simulink model "imusim"  (R2015b)
settings: Solver=FixedStepAuto  StartTime=0.0  StopTime=100  FixedStep=Ts  RelTol=1e-3
values from neighbouring files (symbols this model uses):
  A = quat2mat(q)    [drawframe.m]
  s = sin(theta)    [Phi.m]    (also in ekf_sfun.m = sin(th))
  Ts = 1e-3    (= 0.001)    [setup.m]
undefined symbols (not defined in the file or in its folder): A2, B, B2, X, Y, Z
libraries: sm_lib x12, nesl_utility x8
settings Model: Creator=robots  LastModifiedBy=robots
settings DataIOCC: SaveFormat=Array
settings HardwareCC: ProdBitPerPointer=32  ProdLargestAtomicFloat=None  ProdIntDivRoundTo=Undefined  ProdEndianess=Unspecified  ProdWordSize=32  ProdHWDeviceType=32-bit Generic
settings GRTTargetCC: GeneratePreprocessorConditionals=Disable all
settings ConfigComp: CovModelRefEnable=Off

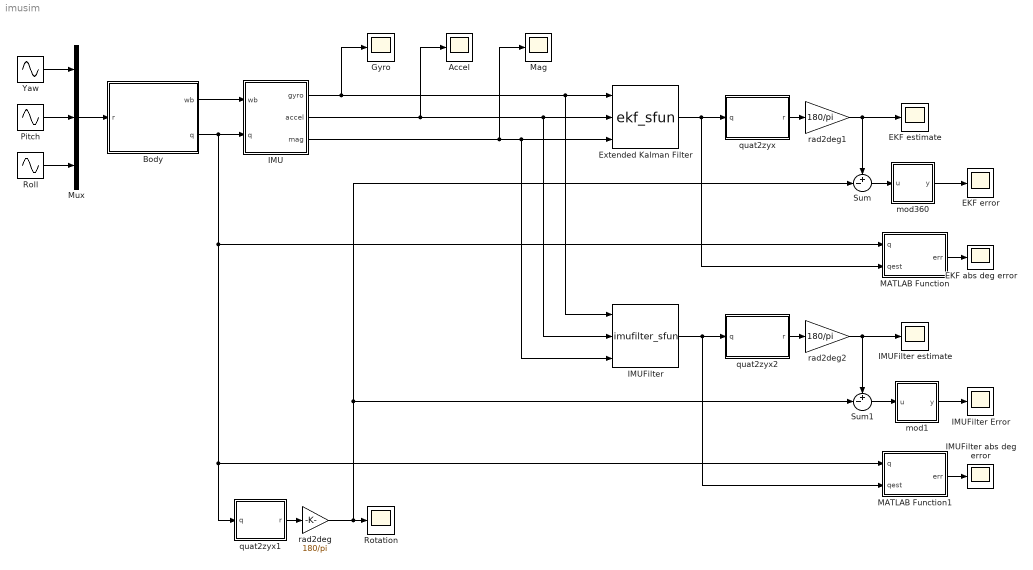
== system imusim ==
  Accel : Scope
  Body : Subsystem
  EKF abs deg error : Scope
  EKF error : Scope
  EKF estimate : Scope
  Extended Kalman Filter : M-S-Function  FunctionName=ekf_sfun  Parameters=Ts, Q, R, gs  mask{Ts=Ts, Q=diag([1 1 1 1]), R=diag([1e6*[1 1 1] 1e8*[1 1 1]]), gs=500/180*pi/2^15}
      mask prompts: Ts "Sample time (-1 for inherited):"; Q "Model covariance matrix (Q):"; R "Measurement covariance matrix (R):"; gs "Rate gyro scale:"
      mask Display:
      | port_label('input', 1, 'gyro')
      | port_label('input', 2, 'accel')
      | port_label('input', 3, 'mag')
      | port_label('output', 1, 'q')
  Gyro : Scope
  IMU : Subsystem
  IMUFilter : M-S-Function  FunctionName=imufilter_sfun  Parameters=Ts, gv, av, mv, gs  mask{Ts=Ts, gv=1, av=1e6, mv=1e8, gs=500/180*pi/2^15}
      mask prompts: Ts "Sample time (-1 for inherited):"; gv "Rate gyro variance:"; av "Accelerometer variance:"; mv "Magnetometer variance:"; gs "Rate gyro scale:"
      mask Display:
      | port_label('input', 1, 'gyro')
      | port_label('input', 2, 'accel')
      | port_label('input', 3, 'mag')
      | port_label('output', 1, 'q')
  IMUFilter abs deg error : Scope
  IMUFilter Error : Scope
  IMUFilter estimate : Scope
  MATLAB Function : MATLAB Function  TreatAsAtomicUnit=on
  MATLAB Function1 : MATLAB Function  TreatAsAtomicUnit=on
  Mag : Scope
  Mux : Mux  Inputs=3
  Pitch : Sin  Amplitude=0.5  Frequency=2*pi  SampleTime=0
  Roll : Sin  Amplitude=0  Frequency=2*pi  SampleTime=0
  Rotation : Scope
  Sum : Sum  Inputs=+-|
  Sum1 : Sum  Inputs=+-|
  Yaw : Sin  Amplitude=0  Frequency=2*pi  SampleTime=0
  mod1 : MATLAB Function  TreatAsAtomicUnit=on
  mod360 : MATLAB Function  TreatAsAtomicUnit=on
  quat2zyx : MATLAB Function  TreatAsAtomicUnit=on
  quat2zyx1 : MATLAB Function  TreatAsAtomicUnit=on
  quat2zyx2 : MATLAB Function  TreatAsAtomicUnit=on
  rad2deg : Gain  Gain=180/pi
  rad2deg1 : Gain  Gain=180/pi
  rad2deg2 : Gain  Gain=180/pi
  wires:
  Extended Kalman Filter/1 -> quat2zyx/1(q), MATLAB Function/2(qest)
  quat2zyx/1(r) -> rad2deg1/1
  Sum/1 -> mod360/1(u)
  mod360/1(y) -> EKF error/1
  MATLAB Function/1(err) -> EKF abs deg error/1
  IMUFilter/1 -> quat2zyx2/1(q), MATLAB Function1/2(qest)
  quat2zyx2/1(r) -> rad2deg2/1
  Sum1/1 -> mod1/1(u)
  mod1/1(y) -> IMUFilter Error/1
  MATLAB Function1/1(err) -> IMUFilter abs deg error/1
  Mux/1 -> Body/1(r)
  Body/1(wb) -> IMU/1(wb)
  Yaw/1 -> Mux/1
  Pitch/1 -> Mux/2
  Roll/1 -> Mux/3
  quat2zyx1/1(r) -> rad2deg/1
  Body/2(q) -> MATLAB Function1/1(q), quat2zyx1/1(q), MATLAB Function/1(q), IMU/2(q)
  rad2deg/1 -> Rotation/1, Sum1/2, Sum/2
  rad2deg1/1 -> EKF estimate/1, Sum/1
  rad2deg2/1 -> Sum1/1, IMUFilter estimate/1
  IMU/1(gyro) -> IMUFilter/1, Extended Kalman Filter/1, Gyro/1
  IMU/3(mag) -> IMUFilter/3, Extended Kalman Filter/3, Mag/1
  IMU/2(accel) -> Accel/1, IMUFilter/2, Extended Kalman Filter/2

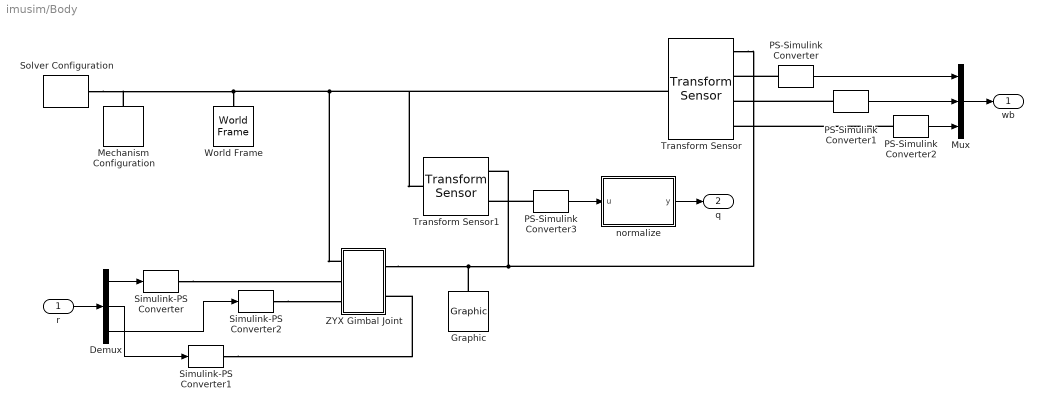
== system imusim/Body ==
  r : Inport
  Demux : Demux  Outputs=3
  Graphic : sm_lib/Body Elements/Graphic  GraphicType=Marker  MarkerShape=Frame  MarkerSize=64  GraphicVisPropType=SimpleVisualProperties  GraphicDiffuseColor=[1.0 0.0 0.0]  GraphicSpecularColor=[0.5 0.5 0.5 1.0]  GraphicAmbientColor=[0.15 0.15 0.15 1.0]  GraphicEmissiveColor=[0.0 0.0 0.0 1.0]  GraphicShininess=75  GraphicOpacity=1.0  BlockFunction=simmechanics.library.body_elements.graphic
  Mechanism Configuration : sm_lib/Utilities/Mechanism Configuration  UniformGravity=Constant  GravityVector=[0 0 -9.80665]  GravityUnits=m/s^2  LinearizationDelta=0.001  BlockFunction=simmechanics.library.utilities.mechanism_configuration
  Mux : Mux  Inputs=3
  PS-Simulink Converter : nesl_utility/PS-Simulink Converter  PhysicalDomain=network_engine_domain  SubClassName=ps_output  LeftPortType=input  RightPortType=output  PseudoPeriodic=off  Frequencies=[]  Unit=rad/s  AffineConversion=off
  PS-Simulink Converter1 : nesl_utility/PS-Simulink Converter  PhysicalDomain=network_engine_domain  SubClassName=ps_output  LeftPortType=input  RightPortType=output  PseudoPeriodic=off  Frequencies=[]  Unit=rad/s  AffineConversion=off
  PS-Simulink Converter2 : nesl_utility/PS-Simulink Converter  PhysicalDomain=network_engine_domain  SubClassName=ps_output  LeftPortType=input  RightPortType=output  PseudoPeriodic=off  Frequencies=[]  Unit=rad/s  AffineConversion=off
  PS-Simulink Converter3 : nesl_utility/PS-Simulink Converter  PhysicalDomain=network_engine_domain  SubClassName=ps_output  LeftPortType=input  RightPortType=output  PseudoPeriodic=off  Frequencies=[]  Unit=1  AffineConversion=off
  Simulink-PS Converter : nesl_utility/Simulink-PS Converter  PhysicalDomain=network_engine_domain  SubClassName=ps_input  LeftPortType=input  RightPortType=output  PseudoPeriodic=off  Frequencies=[]  NoiseDistribution=none  NoiseParameters=[]  Unit=rad  AffineConversion=off  InputFiltering=on  SimscapeFilterOrder=2  InputFilterTimeConstant=0.001  UdotUserProvided=1
  Simulink-PS Converter1 : nesl_utility/Simulink-PS Converter  PhysicalDomain=network_engine_domain  SubClassName=ps_input  LeftPortType=input  RightPortType=output  PseudoPeriodic=off  Frequencies=[]  NoiseDistribution=none  NoiseParameters=[]  Unit=rad  AffineConversion=off  InputFiltering=on  SimscapeFilterOrder=2  InputFilterTimeConstant=0.001  UdotUserProvided=1
  Simulink-PS Converter2 : nesl_utility/Simulink-PS Converter  PhysicalDomain=network_engine_domain  SubClassName=ps_input  LeftPortType=input  RightPortType=output  PseudoPeriodic=off  Frequencies=[]  NoiseDistribution=none  NoiseParameters=[]  Unit=rad  AffineConversion=off  InputFiltering=on  SimscapeFilterOrder=2  InputFilterTimeConstant=0.001  UdotUserProvided=1
  Solver Configuration : nesl_utility/Solver Configuration  PhysicalDomain=network_engine_domain  SubClassName=solver  LeftPortType=input  RightPortType=generic  Accelerate=off  Tones=[]  Harmonics=[]  SimulateNoise=off  Profile=off  UseLocalSampling=off  EnableSwitchedLinearOptims=on  FrequencyDomain=off  UseCCode=off  RelTol=0.001  AbsTol=1e-06  MinStep=1e-09  ToWorkspace=off  RevertToSquareIcSolve=off  NumHomotopyIterations=100  PhasorMode=off  PhasorModeNumHarmonics=1  DoDC=off  ResidualTolerance=1e-09  UseLocalSolver=off  LocalSolverChoice=NE_BACKWARD_EULER_ADVANCER  LocalSolverSampleTime=0.001  DoFixedCost=off  MaxNonlinIter=3  MaxModeIter=2  LinearAlgebra=Sparse  DelaysMemoryBudget=1024  AutomaticFiltering=on  FilteringTimeConstant=0.001
  Transform Sensor : sm_lib/Frames and Transforms/Transform Sensor  MeasurementFrame=Follower  SenseAngle=off  SenseAxis=off  SenseAngle1=off  SenseAngle2=off  SenseAngle3=off  SenseQ=off  SenseR=off  SenseOmegaX=on  SenseOmegaY=on  SenseOmegaZ=on  SenseOmega1=off  SenseOmega2=off  SenseOmega3=off  SenseQDot=off  SenseRDot=off  SenseAlphaX=off  SenseAlphaY=off  SenseAlphaZ=off  SenseAlpha1=off  SenseAlpha2=off  SenseAlpha3=off  SenseQDDot=off  SenseRDDot=off  SenseX=off  SenseY=off  SenseZ=off  SenseRad=off  SenseAzim=off  SenseDist=off  SenseInc=off  SenseXDot=off  SenseYDot=off  SenseZDot=off  SenseRadDot=off  SenseAzimDot=off  SenseDistDot=off  SenseIncDot=off  SenseXDDot=off  SenseYDDot=off  SenseZDDot=off  SenseRadDDot=off  SenseAzimDDot=off  SenseDistDDot=off  SenseIncDDot=off  BlockFunction=simmechanics.library.frames_transforms.transform_sensor
  Transform Sensor1 : sm_lib/Frames and Transforms/Transform Sensor  MeasurementFrame=Base  SenseAngle=off  SenseAxis=off  SenseAngle1=off  SenseAngle2=off  SenseAngle3=off  SenseQ=on  SenseR=off  SenseOmegaX=off  SenseOmegaY=off  SenseOmegaZ=off  SenseOmega1=off  SenseOmega2=off  SenseOmega3=off  SenseQDot=off  SenseRDot=off  SenseAlphaX=off  SenseAlphaY=off  SenseAlphaZ=off  SenseAlpha1=off  SenseAlpha2=off  SenseAlpha3=off  SenseQDDot=off  SenseRDDot=off  SenseX=off  SenseY=off  SenseZ=off  SenseRad=off  SenseAzim=off  SenseDist=off  SenseInc=off  SenseXDot=off  SenseYDot=off  SenseZDot=off  SenseRadDot=off  SenseAzimDot=off  SenseDistDot=off  SenseIncDot=off  SenseXDDot=off  SenseYDDot=off  SenseZDDot=off  SenseRadDDot=off  SenseAzimDDot=off  SenseDistDDot=off  SenseIncDDot=off  BlockFunction=simmechanics.library.frames_transforms.transform_sensor
  World Frame : sm_lib/Frames and Transforms/World Frame  BlockFunction=simmechanics.library.frames_transforms.world_frame
  ZYX Gimbal Joint : Subsystem
  normalize : MATLAB Function  TreatAsAtomicUnit=on
  wb : Outport
  q : Outport  Port=2
  wires:
  Mux/1 -> wb/1
  PS-Simulink Converter/1 -> Mux/1
  PS-Simulink Converter1/1 -> Mux/2
  PS-Simulink Converter2/1 -> Mux/3
  PS-Simulink Converter3/1 -> normalize/1(u)
  Demux/1 -> Simulink-PS Converter/1
  Demux/2 -> Simulink-PS Converter1/1
  Demux/3 -> Simulink-PS Converter2/1
  r/1 -> Demux/1
  normalize/1(y) -> q/1
  connections:
  ZYX Gimbal Joint/RConn1 -- Transform Sensor/RConn1 -- Transform Sensor1/RConn1 -- Graphic/RConn1
  World Frame/RConn1 -- ZYX Gimbal Joint/LConn1 -- Transform Sensor1/LConn1 -- Transform Sensor/LConn1 -- Mechanism Configuration/RConn1 -- Solver Configuration/RConn1
  PS-Simulink Converter/LConn1 -- Transform Sensor/RConn2
  PS-Simulink Converter1/LConn1 -- Transform Sensor/RConn3
  PS-Simulink Converter2/LConn1 -- Transform Sensor/RConn4
  PS-Simulink Converter3/LConn1 -- Transform Sensor1/RConn2
  Simulink-PS Converter/RConn1 -- ZYX Gimbal Joint/LConn2
  Simulink-PS Converter1/RConn1 -- ZYX Gimbal Joint/RConn2
  Simulink-PS Converter2/RConn1 -- ZYX Gimbal Joint/LConn3

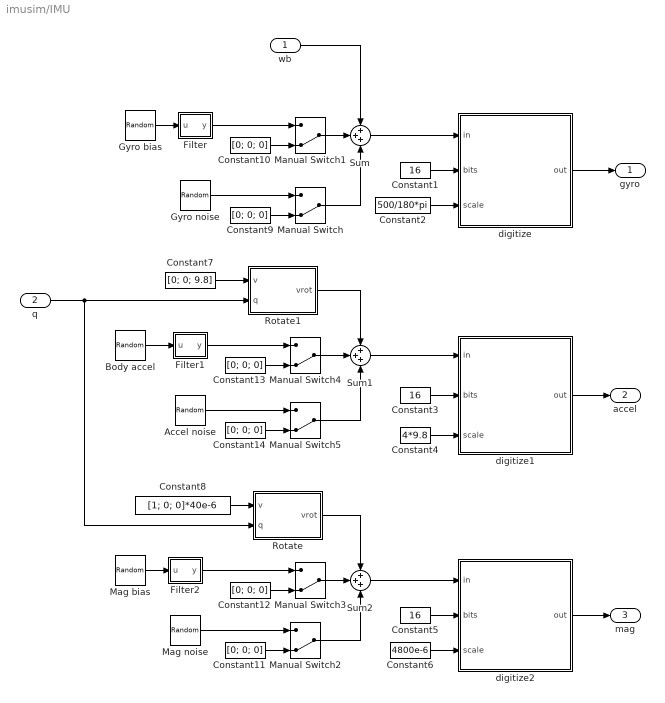
== system imusim/IMU ==
  wb : Inport
  q : Inport  Port=2
  Accel noise : RandomNumber  Variance=(4e-2)^2  Seed=[12 13 14]  SampleTime=Ts
  Body accel : RandomNumber  Variance=(3)^2  Seed=[9 10 11]  SampleTime=1
  Constant1 : Constant  Value=16
  Constant{9..14} (6 alike) : Constant  Value=[0; 0; 0]
  Constant2 : Constant  Value=500/180*pi
  Constant3 : Constant  Value=16
  Constant4 : Constant  Value=4*9.8
  Constant5 : Constant  Value=16
  Constant6 : Constant  Value=4800e-6
  Constant7 : Constant  Value=[0; 0; 9.8]
  Constant8 : Constant  Value=[1; 0; 0]*40e-6
  Filter : Subsystem
  Filter1 : Subsystem
  Filter2 : Subsystem
  Gyro bias : RandomNumber  Variance=(4e-3)^2  Seed=[3 4 5]  SampleTime=20
  Gyro noise : RandomNumber  Variance=(4e-3)^2  Seed=[6 7 8]  SampleTime=Ts
  Mag bias : RandomNumber  Variance=(4e-6)^2  Seed=[15 16 17]  SampleTime=1
  Mag noise : RandomNumber  Variance=(2e-6)^2  Seed=[18 19 20]  SampleTime=Ts
  Manual Switch{,1..5} (6 alike) : ManualSwitch  CurrentSetting=0
  Rotate : MATLAB Function  TreatAsAtomicUnit=on
  Rotate1 : MATLAB Function  TreatAsAtomicUnit=on
  Sum : Sum  Inputs=+++
  Sum1 : Sum  Inputs=+++
  Sum2 : Sum  Inputs=+++
  digitize : MATLAB Function  TreatAsAtomicUnit=on
  digitize1 : MATLAB Function  TreatAsAtomicUnit=on
  digitize2 : MATLAB Function  TreatAsAtomicUnit=on
  gyro : Outport
  accel : Outport  Port=2
  mag : Outport  Port=3
  wires:
  wb/1 -> Sum/1
  Gyro bias/1 -> Filter/1(u)
  Sum/1 -> digitize/1(in)
  Constant1/1 -> digitize/2(bits)
  Constant2/1 -> digitize/3(scale)
  Body accel/1 -> Filter1/1(u)
  Sum1/1 -> digitize1/1(in)
  Constant3/1 -> digitize1/2(bits)
  Constant4/1 -> digitize1/3(scale)
  Mag bias/1 -> Filter2/1(u)
  Sum2/1 -> digitize2/1(in)
  Constant5/1 -> digitize2/2(bits)
  Constant6/1 -> digitize2/3(scale)
  digitize2/1(out) -> mag/1
  Rotate1/1(vrot) -> Sum1/1
  Rotate/1(vrot) -> Sum2/1
  digitize1/1(out) -> accel/1
  digitize/1(out) -> gyro/1
  Manual Switch/1 -> Sum/3
  Gyro noise/1 -> Manual Switch/1
  Constant9/1 -> Manual Switch/2
  Constant10/1 -> Manual Switch1/2
  Manual Switch1/1 -> Sum/2
  Filter/1(y) -> Manual Switch1/1
  Constant11/1 -> Manual Switch2/2
  Constant12/1 -> Manual Switch3/2
  Manual Switch3/1 -> Sum2/2
  Manual Switch2/1 -> Sum2/3
  Filter2/1(y) -> Manual Switch3/1
  Mag noise/1 -> Manual Switch2/1
  Constant13/1 -> Manual Switch4/2
  Manual Switch4/1 -> Sum1/2
  Filter1/1(y) -> Manual Switch4/1
  Constant14/1 -> Manual Switch5/2
  Manual Switch5/1 -> Sum1/3
  Accel noise/1 -> Manual Switch5/1
  Constant7/1 -> Rotate1/1(v)
  Constant8/1 -> Rotate/1(v)
  q/1 -> Rotate/2(q), Rotate1/2(q)

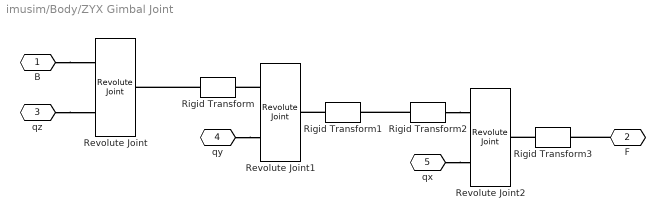
== system imusim/Body/ZYX Gimbal Joint ==
  Revolute Joint : sm_lib/Joints/Revolute Joint  SenseConstraintForce=off  SenseConstraintForceX=off  SenseConstraintForceY=off  SenseConstraintForceZ=off  SenseConstraintTorque=off  SenseConstraintTorqueX=off  SenseConstraintTorqueY=off  SenseConstraintTorqueZ=off  SenseTotalForce=off  SenseTotalForceX=off  SenseTotalForceY=off  SenseTotalForceZ=off  SenseTotalTorque=off  SenseTotalTorqueX=off  SenseTotalTorqueY=off  SenseTotalTorqueZ=off  CompositeWrenchDir=FollowerOnBase  CompositeWrenchFrame=BaseFrame  EquilibriumPosition=0  EquilibriumPositionUnits=deg  SpringStiffness=0  SpringStiffnessUnits=N*m/deg  DampingCoefficient=0  DampingCoefficientUnits=N*m/(deg/s)  TorqueActuationMode=ComputedTorque  MotionActuationMode=InputMotion  SensePosition=off  SenseVelocity=off  SenseAcceleration=off  SenseTorqueForce=off  PositionTargetSpecify=off  PositionTargetPriority=High  PositionTargetValue=0  PositionTargetValueUnits=deg  VelocityTargetSpecify=off  VelocityTargetPriority=High  VelocityTargetValue=0  VelocityTargetValueUnits=deg/s  BlockFunction=simmechanics.library.joints.revolute_joint
  Revolute Joint1 : sm_lib/Joints/Revolute Joint  SenseConstraintForce=off  SenseConstraintForceX=off  SenseConstraintForceY=off  SenseConstraintForceZ=off  SenseConstraintTorque=off  SenseConstraintTorqueX=off  SenseConstraintTorqueY=off  SenseConstraintTorqueZ=off  SenseTotalForce=off  SenseTotalForceX=off  SenseTotalForceY=off  SenseTotalForceZ=off  SenseTotalTorque=off  SenseTotalTorqueX=off  SenseTotalTorqueY=off  SenseTotalTorqueZ=off  CompositeWrenchDir=FollowerOnBase  CompositeWrenchFrame=BaseFrame  EquilibriumPosition=0  EquilibriumPositionUnits=deg  SpringStiffness=0  SpringStiffnessUnits=N*m/deg  DampingCoefficient=0  DampingCoefficientUnits=N*m/(deg/s)  TorqueActuationMode=ComputedTorque  MotionActuationMode=InputMotion  SensePosition=off  SenseVelocity=off  SenseAcceleration=off  SenseTorqueForce=off  PositionTargetSpecify=off  PositionTargetPriority=High  PositionTargetValue=0  PositionTargetValueUnits=deg  VelocityTargetSpecify=off  VelocityTargetPriority=High  VelocityTargetValue=0  VelocityTargetValueUnits=deg/s  BlockFunction=simmechanics.library.joints.revolute_joint
  Revolute Joint2 : sm_lib/Joints/Revolute Joint  SenseConstraintForce=off  SenseConstraintForceX=off  SenseConstraintForceY=off  SenseConstraintForceZ=off  SenseConstraintTorque=off  SenseConstraintTorqueX=off  SenseConstraintTorqueY=off  SenseConstraintTorqueZ=off  SenseTotalForce=off  SenseTotalForceX=off  SenseTotalForceY=off  SenseTotalForceZ=off  SenseTotalTorque=off  SenseTotalTorqueX=off  SenseTotalTorqueY=off  SenseTotalTorqueZ=off  CompositeWrenchDir=FollowerOnBase  CompositeWrenchFrame=BaseFrame  EquilibriumPosition=0  EquilibriumPositionUnits=deg  SpringStiffness=0  SpringStiffnessUnits=N*m/deg  DampingCoefficient=0  DampingCoefficientUnits=N*m/(deg/s)  TorqueActuationMode=ComputedTorque  MotionActuationMode=InputMotion  SensePosition=off  SenseVelocity=off  SenseAcceleration=off  SenseTorqueForce=off  PositionTargetSpecify=off  PositionTargetPriority=High  PositionTargetValue=0  PositionTargetValueUnits=deg  VelocityTargetSpecify=off  VelocityTargetPriority=High  VelocityTargetValue=0  VelocityTargetValueUnits=deg/s  BlockFunction=simmechanics.library.joints.revolute_joint
  Rigid Transform : sm_lib/Frames and Transforms/Rigid Transform  TranslationMethod=None  TranslationLengthUnit=m  TranslationStandardAxis=+Z  TranslationStandardOffset=0  TranslationCartesianOffset=[0 0 0]  TranslationROffset=0  TranslationROffsetUnits=m  TranslationZOffset=0  TranslationZOffsetUnits=m  TranslationThetaOffset=0  TranslationThetaOffsetUnits=deg  RotationMethod=RotationSequence  RotationAngleUnits=deg  RotationStandardAxis=+Z  RotationAngle=0.0  RotationArbitraryAxis=[0 0 1]  FollAlignAxisA=+X  BaseAlignAxisA=+Y  FollAlignAxisB=+Y  BaseAlignAxisB=+Z  RotationSequenceAxes=FollowerAxes  RotationSequence=ZYX  RotationSequenceAngles=[0 0 -90]  RotationSequenceAnglesUnits=deg  RotationMatrix=[1 0 0; 0 1 0; 0 0 1]  BlockFunction=simmechanics.library.frames_transforms.rigid_transform
  Rigid Transform1 : sm_lib/Frames and Transforms/Rigid Transform  TranslationMethod=None  TranslationLengthUnit=m  TranslationStandardAxis=+Z  TranslationStandardOffset=0  TranslationCartesianOffset=[0 0 0]  TranslationROffset=0  TranslationROffsetUnits=m  TranslationZOffset=0  TranslationZOffsetUnits=m  TranslationThetaOffset=0  TranslationThetaOffsetUnits=deg  RotationMethod=RotationSequence  RotationAngleUnits=deg  RotationStandardAxis=+Z  RotationAngle=0.0  RotationArbitraryAxis=[0 0 1]  FollAlignAxisA=+X  BaseAlignAxisA=+Y  FollAlignAxisB=+Y  BaseAlignAxisB=+Z  RotationSequenceAxes=FollowerAxes  RotationSequence=ZYX  RotationSequenceAngles=[0 0 90]  RotationSequenceAnglesUnits=deg  RotationMatrix=[1 0 0; 0 1 0; 0 0 1]  BlockFunction=simmechanics.library.frames_transforms.rigid_transform
  Rigid Transform2 : sm_lib/Frames and Transforms/Rigid Transform  TranslationMethod=None  TranslationLengthUnit=m  TranslationStandardAxis=+Z  TranslationStandardOffset=0  TranslationCartesianOffset=[0 0 0]  TranslationROffset=0  TranslationROffsetUnits=m  TranslationZOffset=0  TranslationZOffsetUnits=m  TranslationThetaOffset=0  TranslationThetaOffsetUnits=deg  RotationMethod=RotationSequence  RotationAngleUnits=deg  RotationStandardAxis=+Z  RotationAngle=0.0  RotationArbitraryAxis=[0 0 1]  FollAlignAxisA=+X  BaseAlignAxisA=+Y  FollAlignAxisB=+Y  BaseAlignAxisB=+Z  RotationSequenceAxes=FollowerAxes  RotationSequence=ZYX  RotationSequenceAngles=[0 90 0]  RotationSequenceAnglesUnits=deg  RotationMatrix=[1 0 0; 0 1 0; 0 0 1]  BlockFunction=simmechanics.library.frames_transforms.rigid_transform
  Rigid Transform3 : sm_lib/Frames and Transforms/Rigid Transform  TranslationMethod=None  TranslationLengthUnit=m  TranslationStandardAxis=+Z  TranslationStandardOffset=0  TranslationCartesianOffset=[0 0 0]  TranslationROffset=0  TranslationROffsetUnits=m  TranslationZOffset=0  TranslationZOffsetUnits=m  TranslationThetaOffset=0  TranslationThetaOffsetUnits=deg  RotationMethod=RotationSequence  RotationAngleUnits=deg  RotationStandardAxis=+Z  RotationAngle=0.0  RotationArbitraryAxis=[0 0 1]  FollAlignAxisA=+X  BaseAlignAxisA=+Y  FollAlignAxisB=+Y  BaseAlignAxisB=+Z  RotationSequenceAxes=FollowerAxes  RotationSequence=ZYX  RotationSequenceAngles=[0 -90 0]  RotationSequenceAnglesUnits=deg  RotationMatrix=[1 0 0; 0 1 0; 0 0 1]  BlockFunction=simmechanics.library.frames_transforms.rigid_transform
  B : PMIOPort  Port=1  Side=Left
  F : PMIOPort  Port=2  Side=Right
  qz : PMIOPort  Port=3  Side=Left
  qy : PMIOPort  Port=4  Side=Right
  qx : PMIOPort  Port=5  Side=Left
  connections:
  Rigid Transform/LConn1 -- Revolute Joint/RConn1
  B/RConn1 -- Revolute Joint/LConn1
  Rigid Transform1/LConn1 -- Revolute Joint1/RConn1
  Revolute Joint1/LConn1 -- Rigid Transform/RConn1
  qz/RConn1 -- Revolute Joint/LConn2
  qy/RConn1 -- Revolute Joint1/LConn2
  Rigid Transform3/LConn1 -- Revolute Joint2/RConn1
  qx/RConn1 -- Revolute Joint2/LConn2
  Rigid Transform2/RConn1 -- Revolute Joint2/LConn1
  Rigid Transform2/LConn1 -- Rigid Transform1/RConn1
  F/RConn1 -- Rigid Transform3/RConn1

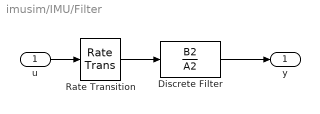
== system imusim/IMU/Filter ==
  u : Inport
  Discrete Filter : DiscreteFilter  Numerator=B2  Denominator=A2
  Rate Transition : RateTransition  OutPortSampleTime=Ts
  y : Outport
  wires:
  u/1 -> Rate Transition/1
  Rate Transition/1 -> Discrete Filter/1
  Discrete Filter/1 -> y/1

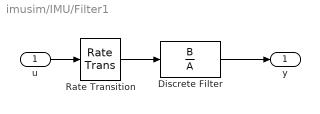
== system imusim/IMU/Filter1 ==
  u : Inport
  Discrete Filter : DiscreteFilter  Numerator=B  Denominator=A
  Rate Transition : RateTransition  OutPortSampleTime=Ts
  y : Outport
  wires:
  u/1 -> Rate Transition/1
  Rate Transition/1 -> Discrete Filter/1
  Discrete Filter/1 -> y/1

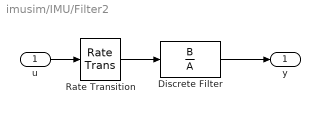
== system imusim/IMU/Filter2 ==
  u : Inport
  Discrete Filter : DiscreteFilter  Numerator=B  Denominator=A
  Rate Transition : RateTransition  OutPortSampleTime=Ts
  y : Outport
  wires:
  u/1 -> Rate Transition/1
  Rate Transition/1 -> Discrete Filter/1
  Discrete Filter/1 -> y/1

== matlab function imusim/IMU/digitize ==
  data: in input; out output; bits input; scale input
function out = digitize(in, bits, scale)
%#codegen

out = floor(min(max(in/scale, -1), 1)*2^(bits-1));

== matlab function imusim/mod360 ==
  data: u input; y output
function y = mod360(u)
%#codegen

y = mod(u + 180, 360) - 180;

== matlab function imusim/IMU/digitize1 ==
  data: in input; out output; bits input; scale input
function out = digitize(in, bits, scale)
%#codegen

out = floor(min(max(in/scale, -1), 1)*2^(bits-1));

== matlab function imusim/IMU/digitize2 ==
  data: in input; out output; bits input; scale input
function out = digitize(in, bits, scale)
%#codegen

out = floor(min(max(in/scale, -1), 1)*2^(bits-1));

== matlab function imusim/IMU/Rotate ==
  data: v input; vrot output; q input
function vrot = rotate(v, q)
%#codegen

vrot = quatrotate(v, quatconj(q));

== matlab function imusim/mod1 ==
  data: u input; y output
function y = mod360(u)
%#codegen

y = mod(u + 180, 360) - 180;

== matlab function imusim/quat2zyx ==
  data: q input; r output
function r = quat2zyx(q)
%#codegen

r = quat2zyx(q);

== matlab function imusim/quat2zyx1 ==
  data: q input; r output
function r = quat2zyx(q)
%#codegen

r = quat2zyx(q);

== matlab function imusim/IMU/Rotate1 ==
  data: v input; vrot output; q input
function vrot = rotate(v, q)
%#codegen

vrot = quatrotate(v, quatconj(q));

== matlab function imusim/MATLAB Function ==
  data: q input; err output; qest input
function err = absdiff(q, qest)
%#codegen

qdiff = quatmul(q, quatconj(qest));
qdiff = qdiff/norm(qdiff);
th = acos(qdiff(1));
err = 2*min(th, pi - th)*180/pi;

== matlab function imusim/MATLAB Function1 ==
  data: q input; err output; qest input
function err = absdiff(q, qest)
%#codegen

qdiff = quatmul(q, quatconj(qest));
qdiff = qdiff/norm(qdiff);
th = acos(qdiff(1));
err = 2*min(th, pi - th)*180/pi;

== matlab function imusim/quat2zyx2 ==
  data: q input; r output
function r = quat2zyx(q)
%#codegen

r = quat2zyx(q);

== matlab function imusim/Body/normalize ==
  data: u input; y output
function y = fcn(u)
%#codegen

y = u/norm(u);
